simulink model "Battery_droop_control_3"  (R2022a)
settings: Solver=ode23tb  StartTime=0.0  StopTime=2  RelTol=1e-3  EnableMultiTasking=on
values from neighbouring files (symbols this model uses):
  R_power_mode_load_change = zeros(1, length(load_percent_list))    [Battery_charge_discharge_FSBB_param_init.m]
  R_voltage_mode_load_change = zeros(1, length(load_percent_list))    [Battery_charge_discharge_FSBB_param_init.m]
  time_step = 1 / wave_freq    (= 2.22222222222e-05)    [Battery_charge_discharge_FSBB_param_init.m]
undefined symbols (not defined in the file or in its folder): Ion, Lithium
libraries: spsSeriesRLCBranchLib x27, spsTriangleGeneratorLib x16, slpidlib x13, spsCurrentMeasurementLib x9, spsIGBTDiodeLib x8, spsIdealSwitchLib x8, spsVoltageMeasurementLib x8, simulink x4, spsBatteryLib x3, spsControlledVoltageSourceLib x3, eeGeneralControl x2, spspowerguiLib x1
(part 4 of 4)

== matlab function Battery_droop_control_3/Battery and DC-DC converter/MATLAB Function ==
  settings: updateMethod=DISCRETE
  data: iL_ref input; u1 output; iL input; vc_ref input; vc input; vin input; i_out input; Ts input; u2 output; Bus_load input
function [u1, u2] = Passivity_BC(iL_ref, iL, vc_ref, vc, vin, i_out, Ts, Bus_load)
% Constant output voltage Module
%   param vc_ref: expected
%   param vc: dcdc output voltage
%   param vin: input voltage
%   param io: current in output side
%   param Bus_load:
%% system parameters
L = 40e-6;  % Inductance 电感 20uH
L_DMinductor = 2.5e-6;
L = L + L_DMinductor;
RL = 0.004;
Co = 2440e-6;  % 电容大小

zeta1 = L / RL * 2000;  % dumping gains
zeta2 = Co * 1000; 

% if Bus_load > 1e4
%     zeta2 = 1e-3;
% end


% error functions: state variable
x1 = iL - iL_ref;
x2 = vc - vc_ref;
persistent iL_ref_old vc_ref_old;
if isempty(iL_ref_old)
    iL_ref_old = 0;
    vc_ref_old = 0;
end

diL_ref = (iL_ref - iL_ref_old) / Ts;
dvc_ref = (vc_ref - vc_ref_old) / Ts;
%% calculate switching signal: u1,u2
% u2 denotes S3's state
% u1 denotes S1's state
u2 = 1 / iL_ref * (iL_ref - dvc_ref * Co - i_out + x2*zeta2);
u1 = 1 / vin * (L*diL_ref + RL*iL_ref + vc_ref*(1-u2) - x1*zeta1);
iL_ref_old = iL_ref;
vc_ref_old = vc_ref;

% compensate strategy
S1_duty_cycle = vc_ref / vin;
S4_duty_cycle = 1 - vin / vc_ref;  % vin < vc
S3_duty_cycle = 1- S4_duty_cycle;
PWM_triangular_wave_range = 2;
PWM_triangular_wave_min = -1;
original_u2 = u2;


persistent voltage_surge_max;
if isempty(voltage_surge_max)
    voltage_surge_max = 0;
end

if Bus_load > 1e2
    u2 = S4_duty_cycle;  % need to check
end


% Modify overshoot at initial stage
if vc - vc_ref > 1 %&& (vc - voltage_surge_max > -0.4)
    u2 = 2;
%     u2 = S3_duty_cycle * PWM_triangular_wave_range + PWM_triangular_wave_min;
    if vin - vc_ref > 1
        u1 = (1 - S1_duty_cycle) * PWM_triangular_wave_range + PWM_triangular_wave_min;
    end
end

% BoostMode
if vc_ref -vc > 0.5 % && Bus_load > 1e2
    u2 = S4_duty_cycle;
%     u2 = S3_duty_cycle * PWM_triangular_wave_range + PWM_triangular_wave_min;
    u1 = max(u1, S3_duty_cycle* PWM_triangular_wave_range + PWM_triangular_wave_min);
%     u1 = 2;
end


if abs(i_out) < 5 && abs(vc - vc_ref) < 0.3
    u2 = S4_duty_cycle;
end




% % Boost mode
% if (vc_ref - vin) > 1 && (vc_ref - vc) > 0.5
%     u1 = S1_duty_cycle * PWM_triangular_wave_range + PWM_triangular_wave_min;
% %     u2 = S4_duty_cycle * PWM_triangular_wave_range + PWM_triangular_wave_min;
% end
% 
% % Buck mode
% if vin - vc_ref > 1 && vc - vc_ref > 1
%     u2 = 2;
% %     u1 = S1_duty_cycle * PWM_triangular_wave_range + PWM_triangular_wave_min;
% end

voltage_surge_max = max(vc, voltage_surge_max);

== matlab function Battery_droop_control_3/Battery and DC-DC converter/MATLAB Function2 ==
  settings: updateMethod=DISCRETE
  data: iL_ref input; u1 output; iL input; i_out_ref input; i_out input; vin input; Vc input; Ts input; u2 output
function [u1, u2] = Passivity_BC(iL_ref, iL,i_out_ref, i_out, vin, Vc, Ts)
% Constant output current Module
% param iL: inductor's current
% param iL_ref: expected value of inductor's current
% param i_out: dcdc output current 
% param i_out_ref
% param vin: input voltage
% param Vc: output voltage
%% system parameters
L = 40e-6;  % Inductance 电感 20uH
L_DMinductor = 2.2e-6;
L = L + L_DMinductor;
RL = 0.004;
C_output = 1440e-6;  % 电容大小

% zeta1 = 6 * 2;  % dumping gains
% zeta2 = 0.08 * 10;
zeta1 = L / RL * 2000;  % dumping gains
zeta2 = C_output * 1000; 

% error functions: state variable
x1 = iL - iL_ref;
x2 = i_out - i_out_ref;
persistent iL_ref_old Vc_old;
if isempty(iL_ref_old)
    iL_ref_old = 0;
    Vc_old = 0;
end

diL_ref = (iL_ref - iL_ref_old) / Ts;
dVc_ref = (Vc - Vc_old) / Ts;
%% calculate switching signal: u1,u2
u2 = 1 / iL_ref * (iL_ref - C_output * dVc_ref - i_out_ref + x2*zeta2);
u1 = 1 / vin * (L*diL_ref + RL * iL_ref + Vc * (1 - u2) - x1*zeta1);

iL_ref_old = iL_ref;
Vc_old = Vc;

== matlab function Battery_droop_control_3/Battery and DC-DC converter/MATLAB Function3 ==
  settings: updateMethod=DISCRETE
  data: iL_ref input; u1 output; iL input; vc_ref input; vc input; vin input; i_out input; Ts input; u2 output
function [u1, u2] = Passivity_BC(iL_ref, iL, vc_ref, vc, vin, i_out, Ts)
% Constant output voltage Module
%   param vc_ref: expected
%   param vc: dcdc output voltage
%   param vin: input voltage
%   param io: current in output side
%% system parameters
L = 2 * 40e-6;  % Inductance 电感 20uH
L_DMinductor = 2.2e-6;
L = L + L_DMinductor;
RL = 0.004;
Co = 1440e-6;  % 电容大小

zeta1 = 6 * 2;  % dumping gains
zeta2 = 0.08 * 10; 

% error functions: state variable
x1 = iL - iL_ref;
x2 = vc - vc_ref;
persistent iL_ref_old vc_ref_old;
if isempty(iL_ref_old)
    iL_ref_old = 0;
    vc_ref_old = 0;
end

diL_ref = (iL_ref - iL_ref_old) / Ts;
dvc_ref = (vc_ref - vc_ref_old) / Ts;
%% calculate switching signal: u1,u2
u2 = 1 / iL_ref * (iL_ref - dvc_ref * Co - i_out + x2*zeta2);
u1 = 1 / vin * (L*diL_ref + RL*iL_ref + vc_ref*(1-u2) - x1*zeta1);
iL_ref_old = iL_ref;
vc_ref_old = vc_ref;

== matlab function Battery_droop_control_3/Battery and DC-DC converter/Discharge Const Voltage/MATLAB Function1 ==
  settings: updateMethod=DISCRETE
  data: iL_ref input; u1 output; iL input; vc_ref input; vc input; vin input; i_out input; Ts input; u2 output; Bus_load input
function [u1, u2] = Passivity_BC(iL_ref, iL, vc_ref, vc, vin, i_out, Ts, Bus_load)
% Constant output voltage Module
%   param vc_ref: expected
%   param vc: dcdc output voltage
%   param vin: input voltage
%   param io: current in output side
%   param Bus_load:
%% system parameters
L = 40e-6;  % Inductance 电感 20uH
L_DMinductor = 2.2e-6;
L = L + L_DMinductor;
RL = 0.004;
Co = 1440e-6;  % 电容大小

zeta1 = L / RL * 2000;  % dumping gains
zeta2 = Co * 1000; 

% if Bus_load > 1e4
%     zeta2 = 1e-3;
% end


% error functions: state variable
x1 = iL - iL_ref;
x2 = vc - vc_ref;
persistent iL_ref_old vc_ref_old;
if isempty(iL_ref_old)
    iL_ref_old = 0;
    vc_ref_old = 0;
end

diL_ref = (iL_ref - iL_ref_old) / Ts;
dvc_ref = (vc_ref - vc_ref_old) / Ts;
%% calculate switching signal: u1,u2
% u2 denotes S3's state
% u1 denotes S1's state
u2 = 1 / iL_ref * (iL_ref - dvc_ref * Co - i_out + x2*zeta2);
u1 = 1 / vin * (L*diL_ref + RL*iL_ref + vc_ref*(1-u2) - x1*zeta1);
iL_ref_old = iL_ref;
vc_ref_old = vc_ref;

% compensate strategy
S1_duty_cycle = vc_ref / vin;
S4_duty_cycle = 1 - vin / vc_ref;  % vin < vc
S3_duty_cycle = 1- S4_duty_cycle;
PWM_triangular_wave_range = 2;
PWM_triangular_wave_min = -1;
original_u2 = u2;


persistent voltage_surge_max;
if isempty(voltage_surge_max)
    voltage_surge_max = 0;
end

if Bus_load > 1e2
    u2 = S4_duty_cycle;  % need to check
end

% if Bus_load > 1e2 && abs(vc - vc_ref) < 0.2
%     u2 = 0.5 * PWM_triangular_wave_range + PWM_triangular_wave_min;
%     u1 = 0.5 * PWM_triangular_wave_range + PWM_triangular_wave_min;
% end

if vc - vc_ref > 1 % && (vc - voltage_surge_max > -0.4)
%     u2 = 2;
    u2 = S3_duty_cycle * PWM_triangular_wave_range + PWM_triangular_wave_min;
end
if vc - vc_ref > 1 && vin - vc_ref > 1
    u1 = (1 - S1_duty_cycle) * PWM_triangular_wave_range + PWM_triangular_wave_min;
end

% solve buck-boost mode: sudden u2=1, keep bucking
if vc_ref -vc > 0.2 && Bus_load > 1e2
    % In buck-boost mode, start boost when vc starts to drop > 0.3V
    u2 = S4_duty_cycle;
    u1 = max(u1, S3_duty_cycle* PWM_triangular_wave_range + PWM_triangular_wave_min);
end

% % Boost mode
% if (vc_ref - vin) > 1 && (vc_ref - vc) > 0.5
%     u1 = S1_duty_cycle * PWM_triangular_wave_range + PWM_triangular_wave_min;
% %     u2 = S4_duty_cycle * PWM_triangular_wave_range + PWM_triangular_wave_min;
% end
% 
% % Buck mode
% if vin - vc_ref > 1 && vc - vc_ref > 1
%     u2 = 2;
% %     u1 = S1_duty_cycle * PWM_triangular_wave_range + PWM_triangular_wave_min;
% end

voltage_surge_max = max(vc, voltage_surge_max);

== matlab function Battery_droop_control_3/Battery and DC-DC converter/Discharge Mixed CurrentPower/MATLAB Function2 ==
  settings: updateMethod=DISCRETE
  data: iL_ref input; u1 output; iL input; i_out_ref input; i_out input; vin input; Vc input; Ts input; u2 output
function [u1, u2] = Passivity_BC(iL_ref, iL,i_out_ref, i_out, vin, Vc, Ts)
% Constant output current Module
% param iL: inductor's current
% param iL_ref: expected value of inductor's current
% param i_out: dcdc output current 
% param i_out_ref
% param vin: input voltage
% param Vc: output voltage
%% system parameters
L = 40e-6;  % Inductance 电感 20uH
L_DMinductor = 2.2e-6;
L = L + L_DMinductor;
RL = 0.004;
C_output = 1440e-6;  % 电容大小

zeta1 = 6*2;  % dumping gains
zeta2 = 0.08*10;

% error functions: state variable
x1 = iL - iL_ref;
x2 = i_out - i_out_ref;
persistent iL_ref_old Vc_old;
if isempty(iL_ref_old)
    iL_ref_old = 0;
    Vc_old = 0;
end

diL_ref = (iL_ref - iL_ref_old) / Ts;
dVc_ref = (Vc - Vc_old) / Ts;
%% calculate switching signal: u1,u2
u2 = 1 / iL_ref * (iL_ref - C_output * dVc_ref - i_out_ref + x2*zeta2);
u1 = 1 / vin * (L*diL_ref + RL * iL_ref + Vc * (1 - u2) - x1*zeta1);

iL_ref_old = iL_ref;
Vc_old = Vc;
